simulink model "ARX_model_and_neural_network"  (Simulink 5.0)
settings: Solver=ode45  StartTime=0.0  StopTime=96  RelTol=1e-3
libraries: neural x7
settings Model: LastModifiedBy=Admin

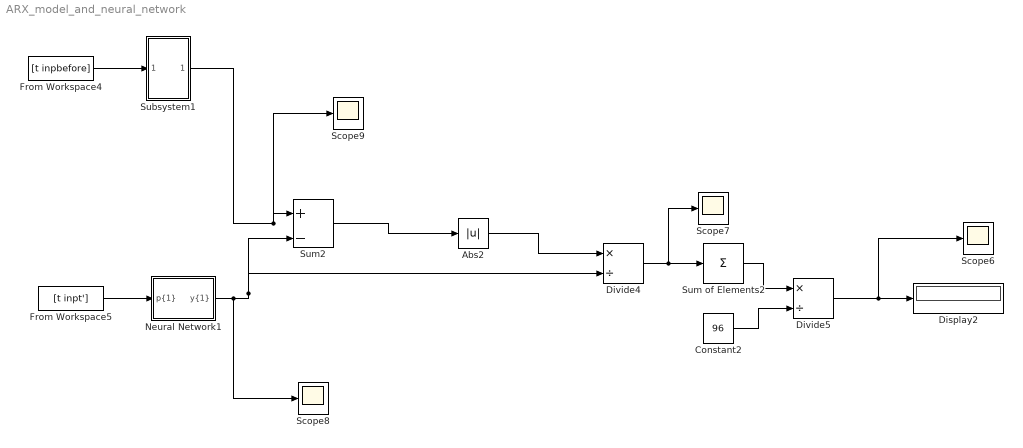
== system ARX_model_and_neural_network ==
  Abs2 : Abs  SaturateOnIntegerOverflow=on
  Constant2 : Constant  Value=96
  Display2 : Display
  Divide4 : Product  Inputs=*/  ShowAdditionalParam=on  OutDataTypeMode=double  OutScaling=2^-10
  Divide5 : Product  Inputs=*/  ShowAdditionalParam=on  OutDataTypeMode=double  OutScaling=2^-10
  From Workspace4 : FromWorkspace  VariableName=[t inpbefore]  SampleTime=0
  From Workspace5 : FromWorkspace  VariableName=[t inpt']  SampleTime=0
  Neural Network1 : Subsystem
  Scope{6..9} (4 alike) : Scope
      Scope8 settings: SaveName=ScopeData2
      Scope9 settings: SaveName=ScopeData3
  Subsystem1 : Subsystem
  Sum of Elements2 : Sum  Inputs=+  ShowAdditionalParam=on  OutDataTypeMode=double  OutScaling=2^-10
  Sum2 : Sum  Inputs=|+-  SaturateOnIntegerOverflow=on
  wires:
  From Workspace5/1 -> Neural Network1/1("p{1}")
  From Workspace4/1 -> Subsystem1/1(In1)
  Sum2/1 -> Abs2/1
  Abs2/1 -> Divide4/1
  Divide4/1 -> Sum of Elements2/1, Scope7/1
  Sum of Elements2/1 -> Divide5/1
  Divide5/1 -> Display2/1, Scope6/1
  Constant2/1 -> Divide5/2
  Subsystem1/1(Out1) -> Sum2/1, Scope9/1
  Neural Network1/1("y{1}") -> Sum2/2, Divide4/2, Scope8/1

== system ARX_model_and_neural_network/Neural Network1 ==
  "p{1}" : Inport  PortDimensions=14  SampleTime=1
  Layer 1 : Subsystem
  Layer 2 : Subsystem
  "y{1}" : Outport  InitialOutput=0
  wires:
  "p{1}"/1 -> Layer 1/1("p{1}")
  Layer 1/1("a{1}") -> [feedback1]
  [feedback1] -> Layer 2/1("a{1} ")
  Layer 2/1("a{2}") -> "y{1}"/1

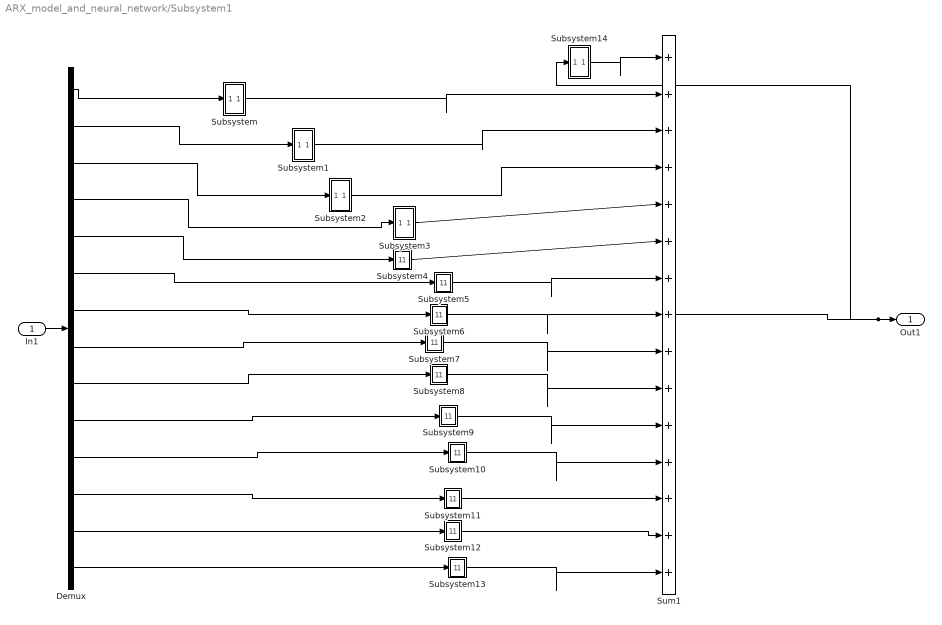
== system ARX_model_and_neural_network/Subsystem1 ==
  In1 : Inport
  Demux : Demux  Outputs=14
  Subsystem : Subsystem
  Subsystem1 : Subsystem
  Subsystem10 : Subsystem
  Subsystem11 : Subsystem
  Subsystem12 : Subsystem
  Subsystem13 : Subsystem
  Subsystem14 : Subsystem
  Subsystem2 : Subsystem
  Subsystem3 : Subsystem
  Subsystem4 : Subsystem
  Subsystem5 : Subsystem
  Subsystem6 : Subsystem
  Subsystem7 : Subsystem
  Subsystem8 : Subsystem
  Subsystem9 : Subsystem
  Sum1 : Sum  Inputs=|+++++++++++++++  SaturateOnIntegerOverflow=on
  Out1 : Outport
  wires:
  Subsystem14/1(Out1) -> Sum1/1
  Sum1/1 -> Subsystem14/1(In1), Out1/1
  Demux/2 -> Subsystem1/1(In1)
  Demux/3 -> Subsystem2/1(In1)
  Demux/4 -> Subsystem3/1(In1)
  Demux/5 -> Subsystem4/1(In1)
  Demux/6 -> Subsystem5/1(In1)
  Demux/7 -> Subsystem6/1(In1)
  Demux/8 -> Subsystem7/1(In1)
  Demux/9 -> Subsystem8/1(In1)
  Demux/10 -> Subsystem9/1(In1)
  Demux/11 -> Subsystem10/1(In1)
  Demux/12 -> Subsystem11/1(In1)
  Demux/13 -> Subsystem12/1(In1)
  Demux/14 -> Subsystem13/1(In1)
  Subsystem13/1(Out1) -> Sum1/15
  Subsystem12/1(Out1) -> Sum1/14
  Subsystem11/1(Out1) -> Sum1/13
  Subsystem10/1(Out1) -> Sum1/12
  Subsystem9/1(Out1) -> Sum1/11
  Subsystem8/1(Out1) -> Sum1/10
  Subsystem7/1(Out1) -> Sum1/9
  Subsystem6/1(Out1) -> Sum1/8
  Subsystem5/1(Out1) -> Sum1/7
  Subsystem4/1(Out1) -> Sum1/6
  Subsystem3/1(Out1) -> Sum1/5
  Subsystem2/1(Out1) -> Sum1/4
  Subsystem1/1(Out1) -> Sum1/3
  Subsystem/1(Out1) -> Sum1/2
  Demux/1 -> Subsystem/1(In1)
  In1/1 -> Demux/1

== system ARX_model_and_neural_network/Neural Network1/Layer 1 ==
  "p{1}" : Inport  PortDimensions=14  SampleTime=1
  Delays 1 : Subsystem
      mask Display: disp('TDL')
  "IW{1,1}" : Subsystem
      mask Display: disp('weight')
  "b{1}" : Constant  Value=[1.7413214757740016;0.69735815383961486;-8.2527879365355368;-3.092693028339442]
      mask Display: disp('bias')
  netsum : Sum  Inputs=2  SaturateOnIntegerOverflow=on  InputSameDT=on
  tansig : neural/Transfer Functions/tansig
  "a{1}" : Outport  InitialOutput=[0;0;0;0]
  wires:
  "p{1}"/1 -> Delays 1/1("p{1}")
  Delays 1/1("pd{1,1}") -> "IW{1,1}"/1("pd{1,1}")
  "IW{1,1}"/1("iz{1,1}") -> netsum/1
  "b{1}"/1 -> netsum/2
  netsum/1 -> tansig/1
  tansig/1 -> "a{1}"/1

== system ARX_model_and_neural_network/Neural Network1/Layer 2 ==
  "a{1} " : Inport  PortDimensions=4  SampleTime=1
  Delays 1 : Subsystem
      mask Display: disp('TDL')
  "LW{2,1}" : Subsystem
      mask Display: disp('weight')
  "b{2}" : Constant  Value=0.82165548242905306
      mask Display: disp('bias')
  netsum : Sum  Inputs=2  SaturateOnIntegerOverflow=on  InputSameDT=on
  tansig : neural/Transfer Functions/tansig
  "a{2}" : Outport  InitialOutput=0
  wires:
  "a{1} "/1 -> Delays 1/1("p{2}")
  Delays 1/1("pd{2,1}") -> "LW{2,1}"/1("ad{2,1}")
  "LW{2,1}"/1("lz{2,1}") -> netsum/1
  "b{2}"/1 -> netsum/2
  netsum/1 -> tansig/1
  tansig/1 -> "a{2}"/1

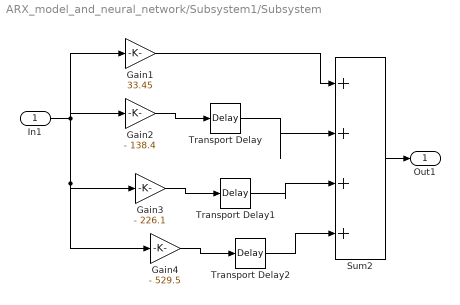
== system ARX_model_and_neural_network/Subsystem1/Subsystem ==
  In1 : Inport
  Gain1 : Gain  Gain=33.45  SaturateOnIntegerOverflow=on
  Gain2 : Gain  Gain=- 138.4  SaturateOnIntegerOverflow=on
  Gain3 : Gain  Gain=- 226.1  SaturateOnIntegerOverflow=on
  Gain4 : Gain  Gain=- 529.5  SaturateOnIntegerOverflow=on
  Sum2 : Sum  Inputs=|++++  SaturateOnIntegerOverflow=on
  Transport Delay : TransportDelay
  Transport Delay1 : TransportDelay  DelayTime=2
  Transport Delay2 : TransportDelay  DelayTime=3
  Out1 : Outport
  wires:
  Gain4/1 -> Transport Delay2/1
  Transport Delay2/1 -> Sum2/4
  Gain2/1 -> Transport Delay/1
  Gain3/1 -> Transport Delay1/1
  Transport Delay/1 -> Sum2/2
  Transport Delay1/1 -> Sum2/3
  Gain1/1 -> Sum2/1
  In1/1 -> Gain2/1, Gain4/1, Gain3/1, Gain1/1
  Sum2/1 -> Out1/1

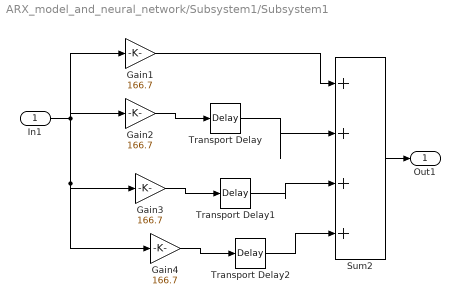
== system ARX_model_and_neural_network/Subsystem1/Subsystem1 ==
  In1 : Inport
  Gain{1..4} (4 alike) : Gain  Gain=166.7  SaturateOnIntegerOverflow=on
  Sum2 : Sum  Inputs=|++++  SaturateOnIntegerOverflow=on
  Transport Delay : TransportDelay
  Transport Delay1 : TransportDelay  DelayTime=2
  Transport Delay2 : TransportDelay  DelayTime=3
  Out1 : Outport
  wires:
  Gain4/1 -> Transport Delay2/1
  Transport Delay2/1 -> Sum2/4
  Gain2/1 -> Transport Delay/1
  Gain3/1 -> Transport Delay1/1
  Transport Delay/1 -> Sum2/2
  Transport Delay1/1 -> Sum2/3
  Gain1/1 -> Sum2/1
  In1/1 -> Gain2/1, Gain4/1, Gain3/1, Gain1/1
  Sum2/1 -> Out1/1

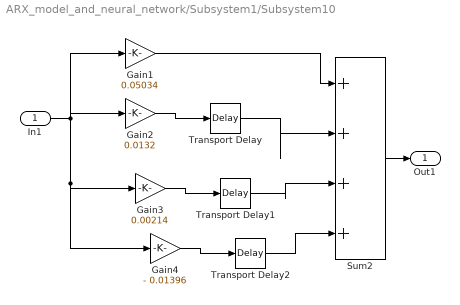
== system ARX_model_and_neural_network/Subsystem1/Subsystem10 ==
  In1 : Inport
  Gain1 : Gain  Gain=0.05034  SaturateOnIntegerOverflow=on
  Gain2 : Gain  Gain=0.0132  SaturateOnIntegerOverflow=on
  Gain3 : Gain  Gain=0.00214  SaturateOnIntegerOverflow=on
  Gain4 : Gain  Gain=- 0.01396  SaturateOnIntegerOverflow=on
  Sum2 : Sum  Inputs=|++++  SaturateOnIntegerOverflow=on
  Transport Delay : TransportDelay
  Transport Delay1 : TransportDelay  DelayTime=2
  Transport Delay2 : TransportDelay  DelayTime=3
  Out1 : Outport
  wires:
  Gain4/1 -> Transport Delay2/1
  Transport Delay2/1 -> Sum2/4
  Gain2/1 -> Transport Delay/1
  Gain3/1 -> Transport Delay1/1
  Transport Delay/1 -> Sum2/2
  Transport Delay1/1 -> Sum2/3
  Gain1/1 -> Sum2/1
  In1/1 -> Gain2/1, Gain4/1, Gain3/1, Gain1/1
  Sum2/1 -> Out1/1

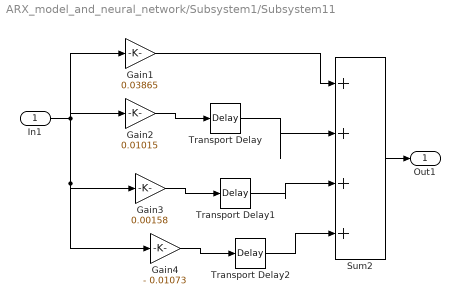
== system ARX_model_and_neural_network/Subsystem1/Subsystem11 ==
  In1 : Inport
  Gain1 : Gain  Gain=0.03865  SaturateOnIntegerOverflow=on
  Gain2 : Gain  Gain=0.01015  SaturateOnIntegerOverflow=on
  Gain3 : Gain  Gain=0.00158  SaturateOnIntegerOverflow=on
  Gain4 : Gain  Gain=- 0.01073  SaturateOnIntegerOverflow=on
  Sum2 : Sum  Inputs=|++++  SaturateOnIntegerOverflow=on
  Transport Delay : TransportDelay
  Transport Delay1 : TransportDelay  DelayTime=2
  Transport Delay2 : TransportDelay  DelayTime=3
  Out1 : Outport
  wires:
  Gain4/1 -> Transport Delay2/1
  Transport Delay2/1 -> Sum2/4
  Gain2/1 -> Transport Delay/1
  Gain3/1 -> Transport Delay1/1
  Transport Delay/1 -> Sum2/2
  Transport Delay1/1 -> Sum2/3
  Gain1/1 -> Sum2/1
  In1/1 -> Gain2/1, Gain4/1, Gain3/1, Gain1/1
  Sum2/1 -> Out1/1

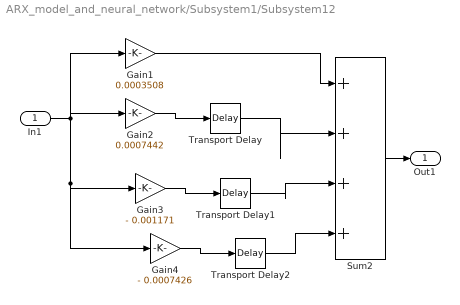
== system ARX_model_and_neural_network/Subsystem1/Subsystem12 ==
  In1 : Inport
  Gain1 : Gain  Gain=0.0003508  SaturateOnIntegerOverflow=on
  Gain2 : Gain  Gain=0.0007442  SaturateOnIntegerOverflow=on
  Gain3 : Gain  Gain=- 0.001171  SaturateOnIntegerOverflow=on
  Gain4 : Gain  Gain=- 0.0007426  SaturateOnIntegerOverflow=on
  Sum2 : Sum  Inputs=|++++  SaturateOnIntegerOverflow=on
  Transport Delay : TransportDelay
  Transport Delay1 : TransportDelay  DelayTime=2
  Transport Delay2 : TransportDelay  DelayTime=3
  Out1 : Outport
  wires:
  Gain4/1 -> Transport Delay2/1
  Transport Delay2/1 -> Sum2/4
  Gain2/1 -> Transport Delay/1
  Gain3/1 -> Transport Delay1/1
  Transport Delay/1 -> Sum2/2
  Transport Delay1/1 -> Sum2/3
  Gain1/1 -> Sum2/1
  In1/1 -> Gain2/1, Gain4/1, Gain3/1, Gain1/1
  Sum2/1 -> Out1/1

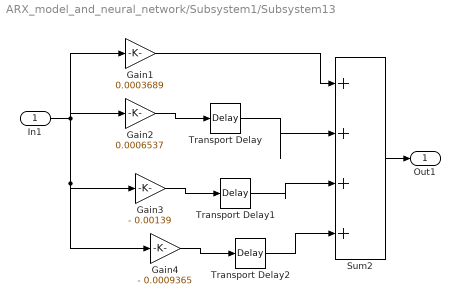
== system ARX_model_and_neural_network/Subsystem1/Subsystem13 ==
  In1 : Inport
  Gain1 : Gain  Gain=0.0003689  SaturateOnIntegerOverflow=on
  Gain2 : Gain  Gain=0.0006537  SaturateOnIntegerOverflow=on
  Gain3 : Gain  Gain=- 0.00139  SaturateOnIntegerOverflow=on
  Gain4 : Gain  Gain=- 0.0009365  SaturateOnIntegerOverflow=on
  Sum2 : Sum  Inputs=|++++  SaturateOnIntegerOverflow=on
  Transport Delay : TransportDelay
  Transport Delay1 : TransportDelay  DelayTime=2
  Transport Delay2 : TransportDelay  DelayTime=3
  Out1 : Outport
  wires:
  Gain4/1 -> Transport Delay2/1
  Transport Delay2/1 -> Sum2/4
  Gain2/1 -> Transport Delay/1
  Gain3/1 -> Transport Delay1/1
  Transport Delay/1 -> Sum2/2
  Transport Delay1/1 -> Sum2/3
  Gain1/1 -> Sum2/1
  In1/1 -> Gain2/1, Gain4/1, Gain3/1, Gain1/1
  Sum2/1 -> Out1/1

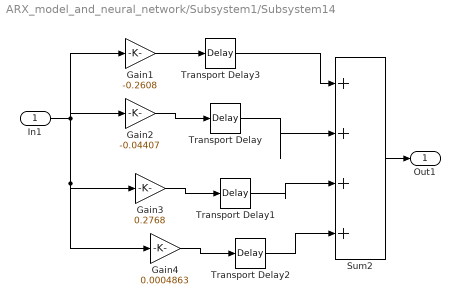
== system ARX_model_and_neural_network/Subsystem1/Subsystem14 ==
  In1 : Inport
  Gain1 : Gain  Gain=-0.2608  SaturateOnIntegerOverflow=on
  Gain2 : Gain  Gain=-0.04407  SaturateOnIntegerOverflow=on
  Gain3 : Gain  Gain=0.2768  SaturateOnIntegerOverflow=on
  Gain4 : Gain  Gain=0.0004863  SaturateOnIntegerOverflow=on
  Sum2 : Sum  Inputs=|++++  SaturateOnIntegerOverflow=on
  Transport Delay : TransportDelay  DelayTime=2
  Transport Delay1 : TransportDelay  DelayTime=3
  Transport Delay2 : TransportDelay  DelayTime=4
  Transport Delay3 : TransportDelay
  Out1 : Outport
  wires:
  Gain4/1 -> Transport Delay2/1
  Transport Delay2/1 -> Sum2/4
  Gain2/1 -> Transport Delay/1
  Gain3/1 -> Transport Delay1/1
  Transport Delay/1 -> Sum2/2
  Transport Delay1/1 -> Sum2/3
  Gain1/1 -> Transport Delay3/1
  In1/1 -> Gain2/1, Gain4/1, Gain3/1, Gain1/1
  Sum2/1 -> Out1/1
  Transport Delay3/1 -> Sum2/1

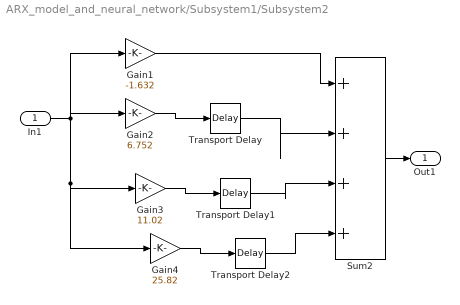
== system ARX_model_and_neural_network/Subsystem1/Subsystem2 ==
  In1 : Inport
  Gain1 : Gain  Gain=-1.632  SaturateOnIntegerOverflow=on
  Gain2 : Gain  Gain=6.752  SaturateOnIntegerOverflow=on
  Gain3 : Gain  Gain=11.02  SaturateOnIntegerOverflow=on
  Gain4 : Gain  Gain=25.82  SaturateOnIntegerOverflow=on
  Sum2 : Sum  Inputs=|++++  SaturateOnIntegerOverflow=on
  Transport Delay : TransportDelay
  Transport Delay1 : TransportDelay  DelayTime=2
  Transport Delay2 : TransportDelay  DelayTime=3
  Out1 : Outport
  wires:
  Gain4/1 -> Transport Delay2/1
  Transport Delay2/1 -> Sum2/4
  Gain2/1 -> Transport Delay/1
  Gain3/1 -> Transport Delay1/1
  Transport Delay/1 -> Sum2/2
  Transport Delay1/1 -> Sum2/3
  Gain1/1 -> Sum2/1
  In1/1 -> Gain2/1, Gain4/1, Gain3/1, Gain1/1
  Sum2/1 -> Out1/1

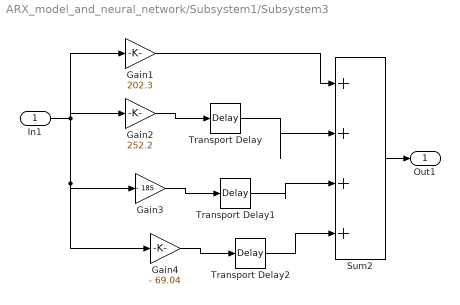
== system ARX_model_and_neural_network/Subsystem1/Subsystem3 ==
  In1 : Inport
  Gain1 : Gain  Gain=202.3  SaturateOnIntegerOverflow=on
  Gain2 : Gain  Gain=252.2  SaturateOnIntegerOverflow=on
  Gain3 : Gain  Gain=- 185  SaturateOnIntegerOverflow=on
  Gain4 : Gain  Gain=- 69.04  SaturateOnIntegerOverflow=on
  Sum2 : Sum  Inputs=|++++  SaturateOnIntegerOverflow=on
  Transport Delay : TransportDelay
  Transport Delay1 : TransportDelay  DelayTime=2
  Transport Delay2 : TransportDelay  DelayTime=3
  Out1 : Outport
  wires:
  Gain4/1 -> Transport Delay2/1
  Transport Delay2/1 -> Sum2/4
  Gain2/1 -> Transport Delay/1
  Gain3/1 -> Transport Delay1/1
  Transport Delay/1 -> Sum2/2
  Transport Delay1/1 -> Sum2/3
  Gain1/1 -> Sum2/1
  In1/1 -> Gain2/1, Gain4/1, Gain3/1, Gain1/1
  Sum2/1 -> Out1/1

== system ARX_model_and_neural_network/Subsystem1/Subsystem4 ==
  In1 : Inport
  Gain1 : Gain  Gain=-200.2  SaturateOnIntegerOverflow=on
  Gain2 : Gain  Gain=- 250.2  SaturateOnIntegerOverflow=on
  Gain3 : Gain  Gain=183.7  SaturateOnIntegerOverflow=on
  Gain4 : Gain  Gain=68.38  SaturateOnIntegerOverflow=on
  Sum2 : Sum  Inputs=|++++  SaturateOnIntegerOverflow=on
  Transport Delay : TransportDelay
  Transport Delay1 : TransportDelay  DelayTime=2
  Transport Delay2 : TransportDelay  DelayTime=3
  Out1 : Outport
  wires:
  Gain4/1 -> Transport Delay2/1
  Transport Delay2/1 -> Sum2/4
  Gain2/1 -> Transport Delay/1
  Gain3/1 -> Transport Delay1/1
  Transport Delay/1 -> Sum2/2
  Transport Delay1/1 -> Sum2/3
  Gain1/1 -> Sum2/1
  In1/1 -> Gain2/1, Gain4/1, Gain3/1, Gain1/1
  Sum2/1 -> Out1/1

== system ARX_model_and_neural_network/Subsystem1/Subsystem5 ==
  In1 : Inport
  Gain1 : Gain  Gain=-1.473  SaturateOnIntegerOverflow=on
  Gain2 : Gain  Gain=- 1.841  SaturateOnIntegerOverflow=on
  Gain3 : Gain  Gain=1.351  SaturateOnIntegerOverflow=on
  Gain4 : Gain  Gain=0.5031  SaturateOnIntegerOverflow=on
  Sum2 : Sum  Inputs=|++++  SaturateOnIntegerOverflow=on
  Transport Delay : TransportDelay
  Transport Delay1 : TransportDelay  DelayTime=2
  Transport Delay2 : TransportDelay  DelayTime=3
  Out1 : Outport
  wires:
  Gain4/1 -> Transport Delay2/1
  Transport Delay2/1 -> Sum2/4
  Gain2/1 -> Transport Delay/1
  Gain3/1 -> Transport Delay1/1
  Transport Delay/1 -> Sum2/2
  Transport Delay1/1 -> Sum2/3
  Gain1/1 -> Sum2/1
  In1/1 -> Gain2/1, Gain4/1, Gain3/1, Gain1/1
  Sum2/1 -> Out1/1

== system ARX_model_and_neural_network/Subsystem1/Subsystem6 ==
  In1 : Inport
  Gain1 : Gain  Gain=-5.55  SaturateOnIntegerOverflow=on
  Gain2 : Gain  Gain=24.53  SaturateOnIntegerOverflow=on
  Gain3 : Gain  Gain=39.93  SaturateOnIntegerOverflow=on
  Gain4 : Gain  Gain=93.38  SaturateOnIntegerOverflow=on
  Sum2 : Sum  Inputs=|++++  SaturateOnIntegerOverflow=on
  Transport Delay : TransportDelay
  Transport Delay1 : TransportDelay  DelayTime=2
  Transport Delay2 : TransportDelay  DelayTime=3
  Out1 : Outport
  wires:
  Gain4/1 -> Transport Delay2/1
  Transport Delay2/1 -> Sum2/4
  Gain2/1 -> Transport Delay/1
  Gain3/1 -> Transport Delay1/1
  Transport Delay/1 -> Sum2/2
  Transport Delay1/1 -> Sum2/3
  Gain1/1 -> Sum2/1
  In1/1 -> Gain2/1, Gain4/1, Gain3/1, Gain1/1
  Sum2/1 -> Out1/1

== system ARX_model_and_neural_network/Subsystem1/Subsystem7 ==
  In1 : Inport
  Gain1 : Gain  Gain=0.0005023  SaturateOnIntegerOverflow=on
  Gain2 : Gain  Gain=- 0.0002562  SaturateOnIntegerOverflow=on
  Gain3 : Gain  Gain=0.0004082  SaturateOnIntegerOverflow=on
  Gain4 : Gain  Gain=- 0.0002853  SaturateOnIntegerOverflow=on
  Sum2 : Sum  Inputs=|++++  SaturateOnIntegerOverflow=on
  Transport Delay : TransportDelay
  Transport Delay1 : TransportDelay  DelayTime=2
  Transport Delay2 : TransportDelay  DelayTime=3
  Out1 : Outport
  wires:
  Gain4/1 -> Transport Delay2/1
  Transport Delay2/1 -> Sum2/4
  Gain2/1 -> Transport Delay/1
  Gain3/1 -> Transport Delay1/1
  Transport Delay/1 -> Sum2/2
  Transport Delay1/1 -> Sum2/3
  Gain1/1 -> Sum2/1
  In1/1 -> Gain2/1, Gain4/1, Gain3/1, Gain1/1
  Sum2/1 -> Out1/1

== system ARX_model_and_neural_network/Subsystem1/Subsystem8 ==
  In1 : Inport
  Gain1 : Gain  Gain=0.0003028  SaturateOnIntegerOverflow=on
  Gain2 : Gain  Gain=0.0008254  SaturateOnIntegerOverflow=on
  Gain3 : Gain  Gain=- 0.0006172  SaturateOnIntegerOverflow=on
  Gain4 : Gain  Gain=0.0001375  SaturateOnIntegerOverflow=on
  Sum2 : Sum  Inputs=|++++  SaturateOnIntegerOverflow=on
  Transport Delay : TransportDelay
  Transport Delay1 : TransportDelay  DelayTime=2
  Transport Delay2 : TransportDelay  DelayTime=3
  Out1 : Outport
  wires:
  Gain4/1 -> Transport Delay2/1
  Transport Delay2/1 -> Sum2/4
  Gain2/1 -> Transport Delay/1
  Gain3/1 -> Transport Delay1/1
  Transport Delay/1 -> Sum2/2
  Transport Delay1/1 -> Sum2/3
  Gain1/1 -> Sum2/1
  In1/1 -> Gain2/1, Gain4/1, Gain3/1, Gain1/1
  Sum2/1 -> Out1/1

== system ARX_model_and_neural_network/Subsystem1/Subsystem9 ==
  In1 : Inport
  Gain1 : Gain  Gain=-0.006094  SaturateOnIntegerOverflow=on
  Gain2 : Gain  Gain=- 0.001589  SaturateOnIntegerOverflow=on
  Gain3 : Gain  Gain=- 0.0002712  SaturateOnIntegerOverflow=on
  Gain4 : Gain  Gain=0.001686  SaturateOnIntegerOverflow=on
  Sum2 : Sum  Inputs=|++++  SaturateOnIntegerOverflow=on
  Transport Delay : TransportDelay
  Transport Delay1 : TransportDelay  DelayTime=2
  Transport Delay2 : TransportDelay  DelayTime=3
  Out1 : Outport
  wires:
  Gain4/1 -> Transport Delay2/1
  Transport Delay2/1 -> Sum2/4
  Gain2/1 -> Transport Delay/1
  Gain3/1 -> Transport Delay1/1
  Transport Delay/1 -> Sum2/2
  Transport Delay1/1 -> Sum2/3
  Gain1/1 -> Sum2/1
  In1/1 -> Gain2/1, Gain4/1, Gain3/1, Gain1/1
  Sum2/1 -> Out1/1

== system ARX_model_and_neural_network/Neural Network1/Layer 1/Delays 1 ==
  "p{1}" : Inport  Orientation=down  PortDimensions=14  SampleTime=1
  mux : Mux  Inputs=1
  "pd{1,1}" : Outport
  wires:
  "p{1}"/1 -> mux/1
  mux/1 -> "pd{1,1}"/1

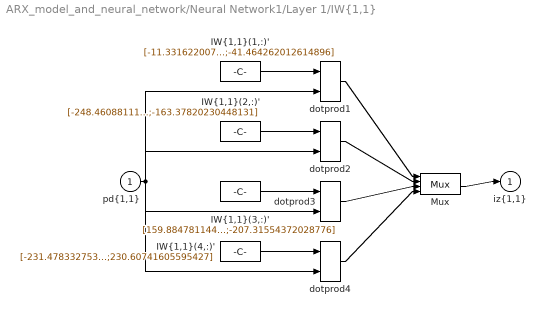
== system ARX_model_and_neural_network/Neural Network1/Layer 1/IW{1,1} ==
  "pd{1,1}" : Inport  PortDimensions=14  SampleTime=1
  "IW{1,1}(1,:)'" : Constant  Value=[-11.331622007191116;480.76986123522266;-244.71826066692819;-215.36506776781869;117.68500710328458;961.37104772765292;-164.93584774087921;-123.71162401167672;-325.39584551772799;869.37046720143348;162.2602095339715;243.93099518166414;250.59760510926006;-41.464262012614896]
      mask Display: disp('weights')
  "IW{1,1}(2,:)'" : Constant  Value=[-248.46088111977173;592.96489870194205;-169.99826511296075;6.7210352268005842;-479.55640228789809;-945.29091142723746;-127.8654249967985;-4.8660732727339644;-66.740410653909109;-1194.9112669366377;-592.82533601042496;-973.13653211376027;-59.240012956465101;-163.37820230448131]
      mask Display: disp('weights')
  "IW{1,1}(3,:)'" : Constant  Value=[159.88478114481589;510.1389358159833;-666.21169528304029;122.42329706388527;73.862813450675262;1057.5895380083077;83.172587324821478;-83.831737188744668;-130.97395062127208;-1449.259370525705;-445.13943115786509;-243.29810900368994;-218.09638607845807;-207.31554372028776]
      mask Display: disp('weights')
  "IW{1,1}(4,:)'" : Constant  Value=[-231.47833275364465;432.94058782940772;481.12543704920199;-189.06868666119615;108.88512919705389;634.60855022269948;33.238156784438438;-420.44459886676248;-87.906302700763874;457.34879761095931;-361.47211045958676;296.27717948861425;-94.358408155950343;230.60741605595427]
      mask Display: disp('weights')
  Mux : Mux
  dotprod{1..4} (4 alike) : neural/Weight Functions/dotprod
  "iz{1,1}" : Outport
  wires:
  "IW{1,1}(1,:)'"/1 -> dotprod1/1
  "pd{1,1}"/1 -> dotprod1/2, dotprod2/2, dotprod3/2, dotprod4/2
  dotprod1/1 -> Mux/1
  "IW{1,1}(2,:)'"/1 -> dotprod2/1
  dotprod2/1 -> Mux/2
  "IW{1,1}(3,:)'"/1 -> dotprod3/1
  dotprod3/1 -> Mux/3
  "IW{1,1}(4,:)'"/1 -> dotprod4/1
  dotprod4/1 -> Mux/4
  Mux/1 -> "iz{1,1}"/1

== system ARX_model_and_neural_network/Neural Network1/Layer 2/Delays 1 ==
  "p{2}" : Inport  Orientation=down  PortDimensions=4  SampleTime=1
  mux : Mux  Inputs=1
  "pd{2,1}" : Outport
  wires:
  "p{2}"/1 -> mux/1
  mux/1 -> "pd{2,1}"/1

== system ARX_model_and_neural_network/Neural Network1/Layer 2/LW{2,1} ==
  "ad{2,1}" : Inport  PortDimensions=4  SampleTime=1
  "IW{2,1}(1,:)'" : Constant  Value=[-0.85082147972736011;-0.0020020092638200438;0.0014643763862159755;-0.038719568952694274]
      mask Display: disp('weights')
  Mux : Mux  Inputs=1
  dotprod1 : neural/Weight Functions/dotprod
  "lz{2,1}" : Outport
  wires:
  "IW{2,1}(1,:)'"/1 -> dotprod1/1
  "ad{2,1}"/1 -> dotprod1/2
  dotprod1/1 -> Mux/1
  Mux/1 -> "lz{2,1}"/1
